simulink model "mux4to1with2to"  (R2024a)
settings: Solver=VariableStepAuto  StartTime=0.0  StopTime=10.0  RelTol=1e-3
settings Model: Creator=tusha  LastModifiedBy=tusha

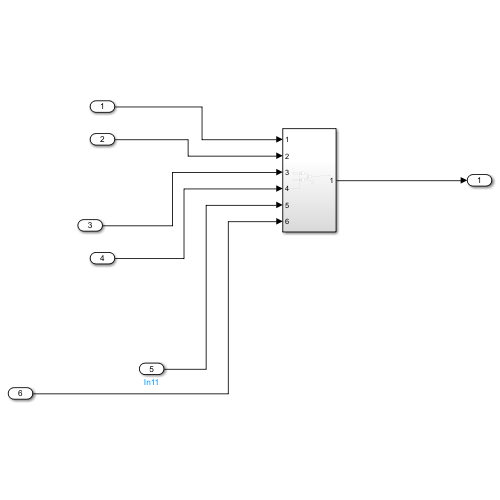
[thumbnail: Simulink's stored preview of the top-level diagram]
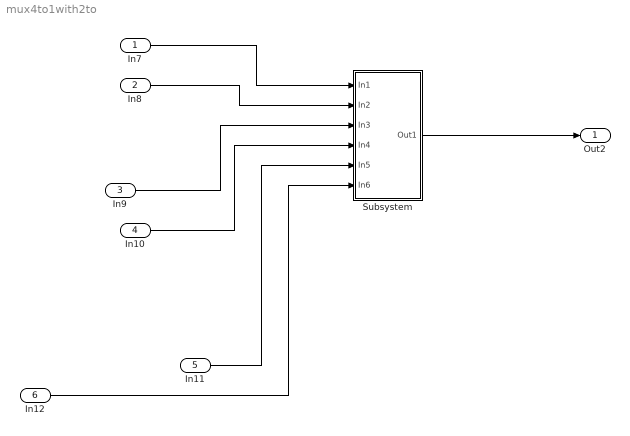
== system mux4to1with2to ==
  In7 : Inport
  In8 : Inport  Port=2
  In9 : Inport  Port=3
  In10 : Inport  Port=4
  In11 : Inport  Port=5
  In12 : Inport  Port=6
  Subsystem : Subsystem
  Out2 : Outport
  wires:
  In7/1 -> Subsystem/1(In1)
  In8/1 -> Subsystem/2(In2)
  In9/1 -> Subsystem/3(In3)
  In10/1 -> Subsystem/4(In4)
  In11/1 -> Subsystem/5(In5)
  In12/1 -> Subsystem/6(In6)
  Subsystem/1(Out1) -> Out2/1

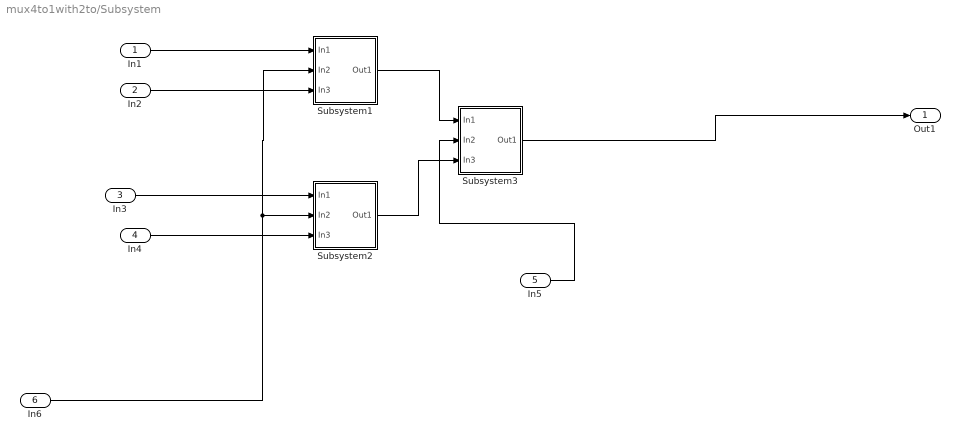
== system mux4to1with2to/Subsystem ==
  In1 : Inport
  In2 : Inport  Port=2
  In3 : Inport  Port=3
  In4 : Inport  Port=4
  In5 : Inport  Port=5
  In6 : Inport  Port=6
  Subsystem1 : Subsystem
  Subsystem2 : Subsystem
  Subsystem3 : Subsystem
  Out1 : Outport
  wires:
  In6/1 -> Subsystem1/2(In2), Subsystem2/2(In2)
  In2/1 -> Subsystem1/3(In3)
  In3/1 -> Subsystem2/1(In1)
  Subsystem2/1(Out1) -> Subsystem3/3(In3)
  Subsystem1/1(Out1) -> Subsystem3/1(In1)
  In4/1 -> Subsystem2/3(In3)
  In1/1 -> Subsystem1/1(In1)
  In5/1 -> Subsystem3/2(In2)
  Subsystem3/1(Out1) -> Out1/1

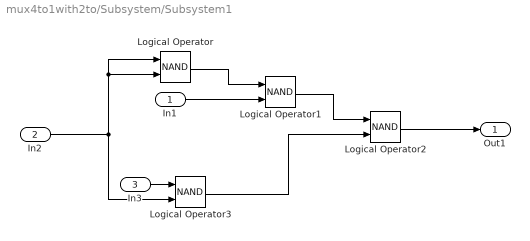
== system mux4to1with2to/Subsystem/Subsystem1 ==
  In1 : Inport
  In2 : Inport  Port=2
  In3 : Inport  Port=3
  Logical Operator{,1..3} (4 alike) : Logic  Operator=NAND  AllPortsSameDT=off  OutDataTypeStr=boolean
  Out1 : Outport
  wires:
  Logical Operator2/1 -> Out1/1
  Logical Operator/1 -> Logical Operator1/1
  In2/1 -> Logical Operator/2, Logical Operator/1, Logical Operator3/2
  Logical Operator1/1 -> Logical Operator2/1
  In1/1 -> Logical Operator1/2
  Logical Operator3/1 -> Logical Operator2/2
  In3/1 -> Logical Operator3/1

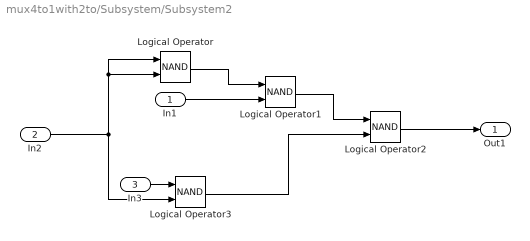
== system mux4to1with2to/Subsystem/Subsystem2 ==
  In1 : Inport
  In2 : Inport  Port=2
  In3 : Inport  Port=3
  Logical Operator{,1..3} (4 alike) : Logic  Operator=NAND  AllPortsSameDT=off  OutDataTypeStr=boolean
  Out1 : Outport
  wires:
  Logical Operator2/1 -> Out1/1
  Logical Operator/1 -> Logical Operator1/1
  In2/1 -> Logical Operator/2, Logical Operator/1, Logical Operator3/2
  Logical Operator1/1 -> Logical Operator2/1
  In1/1 -> Logical Operator1/2
  Logical Operator3/1 -> Logical Operator2/2
  In3/1 -> Logical Operator3/1

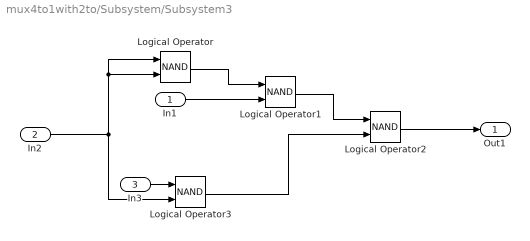
== system mux4to1with2to/Subsystem/Subsystem3 ==
  In1 : Inport
  In2 : Inport  Port=2
  In3 : Inport  Port=3
  Logical Operator{,1..3} (4 alike) : Logic  Operator=NAND  AllPortsSameDT=off  OutDataTypeStr=boolean
  Out1 : Outport
  wires:
  Logical Operator2/1 -> Out1/1
  Logical Operator/1 -> Logical Operator1/1
  In2/1 -> Logical Operator/2, Logical Operator/1, Logical Operator3/2
  Logical Operator1/1 -> Logical Operator2/1
  In1/1 -> Logical Operator1/2
  Logical Operator3/1 -> Logical Operator2/2
  In3/1 -> Logical Operator3/1
